simulink model "simple_coffee"  (R2022a)
settings: Solver=VariableStepAuto  StartTime=0.0  StopTime=10.0  RelTol=1e-3
settings Model: Creator=rmahmoo  LastModifiedBy=rmahmoo

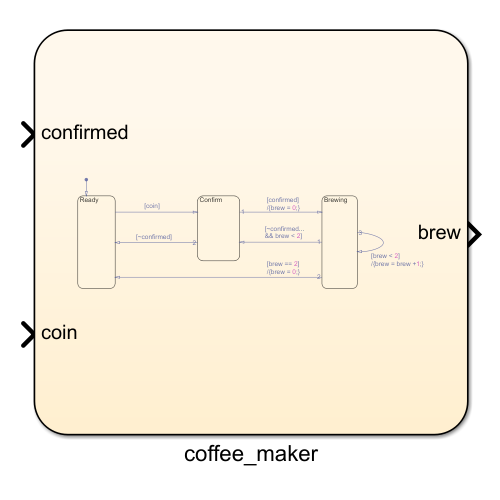
[thumbnail: Simulink's stored preview of the top-level diagram]
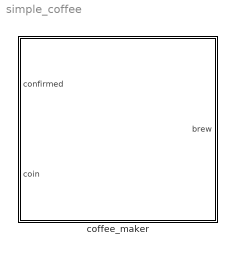
== system simple_coffee ==
  coffee_maker : Stateflow chart  TreatAsAtomicUnit=on

== stateflow chart simple_coffee/coffee_maker ==
  state System
    state Brewer [parallel]
      settings: executionOrder=1
      state Ready
      state Confirm
      state Brewing
      (default) -> Ready
      Ready -> Confirm : [coin]
      Confirm -> Brewing [order 1] : [confirmed]
          | /{brew = 0;}
      Brewing -> Brewing [order 3] : [brew < 2]
          | /{brew = brew +1;}
      Brewing -> Confirm [order 1] : [~confirmed...
          | && brew < 2]
      Confirm -> Ready [order 2] : [~confirmed]
      Brewing -> Ready [order 2] : [brew == 2]
          | /{brew = 0;}
    state Payment [parallel]
      settings: executionOrder=2
      state Idle
      state Paid
      (default) -> Idle
      Paid -> Idle : [confirmed]
      Idle -> Paid : [coin]
  (default) -> System
  data: confirmed input boolean; coin input boolean; brew output uint8 [0..20] =uint8(0)
